simulink model "QPSK_short_4_tx_with_interference"  (R2023a)
settings: Solver=FixedStepAuto  StartTime=0.0  StopTime=inf  RelTol=1e-3
values from neighbouring files (symbols this model uses):
  fs_noise = 2*0.3e6    (= 600000)    [init_parameters_4_tx.m]
  Tx_Antennas = phased.ULA('NumElements',4,'ElementSpacing',0.05,'ArrayAxis','y')    [init_parameters_4_tx.m]
undefined symbols (not defined in the file or in its folder): physconst, qpsktxrx
libraries: dspmathops x4, dspsrcs4 x4, simulink x3, phasedtxrxlib x3, commdigbbndpm3 x3, dspsigops x3, commrflib2 x2, phasedbflib x2, commrfcorlib x2, dspstat3 x2, commsequence2 x2, commsync2 x2
settings Model: SimulationMode=accelerator  Creator=memre  LastModifiedBy=memre
settings DebuggingCC: ParameterOverflowMsg=none  ParameterUnderflowMsg=error

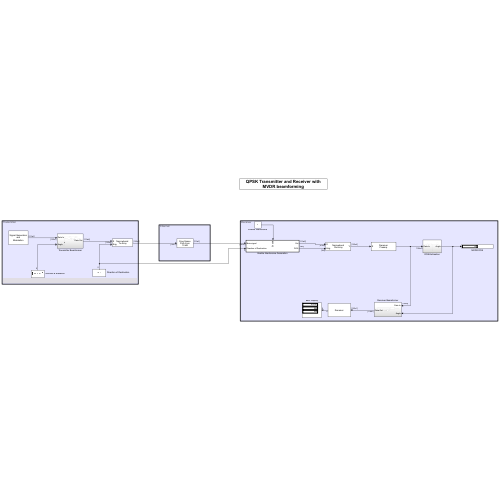
[thumbnail: Simulink's stored preview of the top-level diagram]
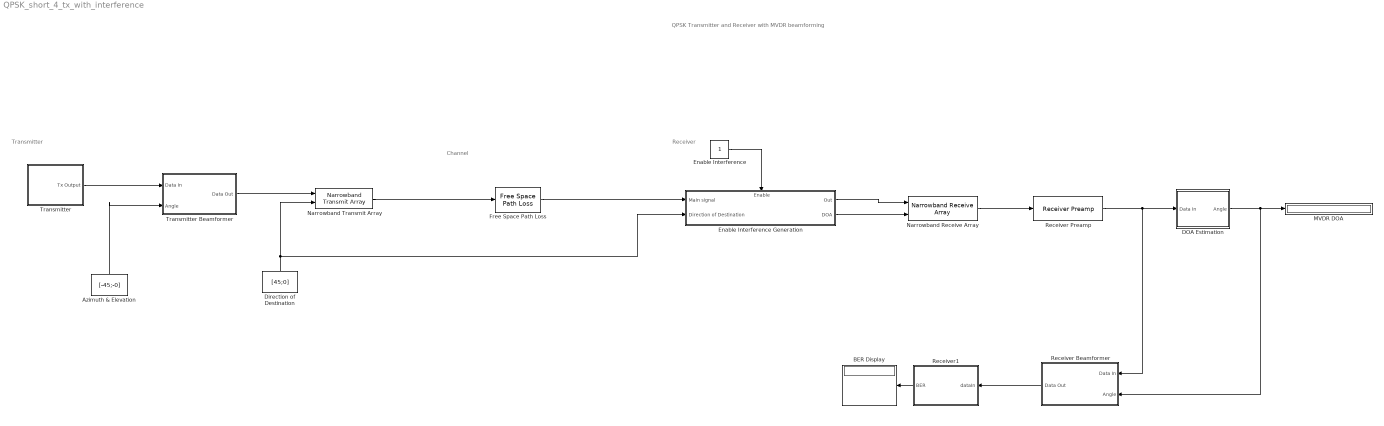
== system QPSK_short_4_tx_with_interference ==
  note: Receiver
  note: Transmitter
  note: Channel
  note: QPSK Transmitter and Receiver with MVDR beamforming
  Azimuth & Elevation : Constant  Value=[-45;-0]
  BER Display : Display
  DOA Estimation : Subsystem
  Direction of Destination : Constant  Value=[45;0]
  Enable Interference : Constant
  Enable Interference Generation : Subsystem  TreatAsAtomicUnit=on
      settings: PortSchema="{\"entries\":[{\"content\":{\"sides\":[{\"content\":{\"connectorIds\":[\"In1\",\"In2\"]},\"type\":\"ConnectorPlacement.EquallySpacedRectSide\",\"uuid\":\"34131771-bf07-4a9f-9b92-1cd845beac1b\"},{\"content\":{\"connectorIds\":[\"Out1\",\"Out2\"],\"side\":\"RIGHT\"},\"type\":\"ConnectorPlacement.EquallySpacedRectSide\",\"uuid\":\"139290bf-3e69-441d-8c76-d9406655bece\"},{\"content\":{\"connectorIds\":[\"In3\"],\"side\":\"TOP\"},\"type\":\"ConnectorPlacement.EquallySpacedRectSide\",\"uuid\":\"20149619-9d5d-4f55-89c0-ec473a07d659\"}]},\"type\":\"ConnectorPlacement.EquallySpacedConnector\",\"uuid\":\"f87a52e8-a08c-4e06-bc9a-bfdf8366a36e\"}],\"packageUris\":[\"http://schema.mathworks.com/mf0/Connector/R2020b\"],\"version\":\"1.0\"}"
  Free Space Path Loss : commrflib2/Free Space Path Loss  mode=Decibels  dB=10  d=0.100  fc=1920
  MVDR DOA : Display
  Narrowband Receive Array : phasedtxrxlib/Narrowband Receive Array  PropagationSpeed=prop_speed  OperatingFrequency=fc  Wavefront=Plane  SensorGainMeasure=dB  Polarization=None  WeightsInputPort=off  SimulateUsing=Interpreted execution  Sensor=Rx_Antennas
  Narrowband Transmit Array : phasedtxrxlib/Narrowband Transmit Array  PropagationSpeed=physconst( 'LightSpeed' )  OperatingFrequency=fc  CombineRadiatedSignals=on  SensorGainMeasure=dB  Polarization=None  WeightsInputPort=off  SimulateUsing=Code generation  Sensor=Tx_Antennas
  Receiver Beamformer : Subsystem
  Receiver Preamp : phasedtxrxlib/Receiver Preamp  Gain=0  LossFactor=0  NoiseMethod=Noise power  NoiseFigure=0  ReferenceTemperature=290  SampleRateFromInputCheckbox=on  SampleRate=1e6  NoisePower=.01  EnableInputPort=off  PhaseNoiseInputPort=off  SeedSource=Auto  Seed=0  SimulateUsing=Interpreted execution
  Receiver1 : Subsystem
      mask Display: disp('Receiver')
  Transmitter : Subsystem
      mask Display: disp('Signal Generation\nand\nModulation')
  Transmitter Beamformer : Subsystem
  wires:
  Receiver1/1(BER) -> BER Display/1
  Direction of Destination/1 -> Enable Interference Generation/2(Direction of Destination), Narrowband Transmit Array/2
  Narrowband Transmit Array/1 -> Free Space Path Loss/1
  Narrowband Receive Array/1 -> Receiver Preamp/1
  Receiver Preamp/1 -> Receiver Beamformer/1(Data In), DOA Estimation/1(Data In)
  Free Space Path Loss/1 -> Enable Interference Generation/1(Main signal)
  Enable Interference/1 -> Enable Interference Generation/3(Enable)
  Enable Interference Generation/1(Out) -> Narrowband Receive Array/1
  Enable Interference Generation/2(DOA) -> Narrowband Receive Array/2
  Transmitter/1(Tx Output) -> Transmitter Beamformer/1(Data In)
  Azimuth & Elevation/1 -> Transmitter Beamformer/2(Angle)
  Transmitter Beamformer/1(Data Out) -> Narrowband Transmit Array/1
  DOA Estimation/1(Angle) -> Receiver Beamformer/2(Angle), MVDR DOA/1
  Receiver Beamformer/1(Data Out) -> Receiver1/1(dataIn)

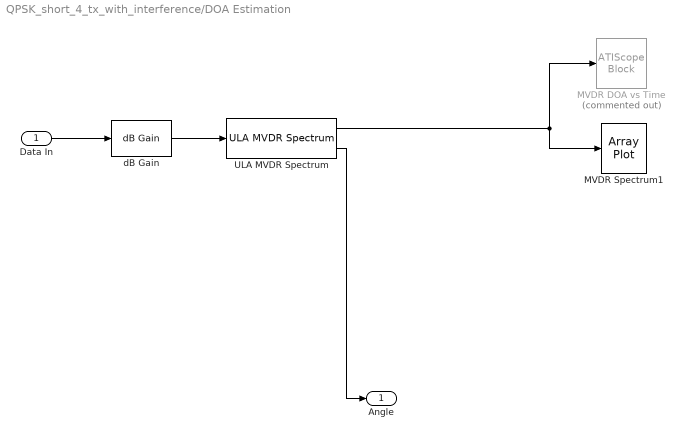
== system QPSK_short_4_tx_with_interference/DOA Estimation ==
  Data In : Inport
  MVDR DOA vs Time : ATIScopeBlock  Commented=on  WindowPosition=[64.000000,127.000000,669.000000,551.000000,]  ScopeFrameLocation=window  AngleLabel=Azimuth Angles (degree)  Title=Angle of Arrival vs. Time  TimeSpan=600  TimeResolution=0.3  ColorbarLabel=magnitude (V)  TimeResolutionSource=Property  TimeSpanSource=Property
  MVDR Spectrum1 : ArrayPlot  WindowPosition=[121.000000,272.000000,887.000000,614.000000,]  ScopeFrameLocation=window  XOffset=10  PlotType=Line  AxesScaling=Manual  Title=MVDR Spectrum  XLabel=Angle (degrees)  YLabel=Magnitude  YLimits=[-1,10]  ShowLegend=on  DefaultConfigurationName=dsp.scopes.ArrayPlotBlockSpecification
  ULA MVDR Spectrum : phaseddoalib/ULA MVDR Spectrum  PropagationSpeed=prop_speed  OperatingFrequency=fc  NumPhaseShifterBits=0  ForwardBackwardAveraging=off  SpatialSmoothing=0  ScanAngles=-90:90  DOAOutputPort=on  NumSignals=1  SimulateUsing=Interpreted execution  SensorArray=Rx_Antennas
  dB Gain : dspmathops/dB Gain  dB=20  intype=Amplitude
  Angle : Outport
  wires:
  ULA MVDR Spectrum/2 -> Angle/1
  ULA MVDR Spectrum/1 -> MVDR Spectrum1/1, MVDR DOA vs Time/1
  Data In/1 -> dB Gain/1
  dB Gain/1 -> ULA MVDR Spectrum/1

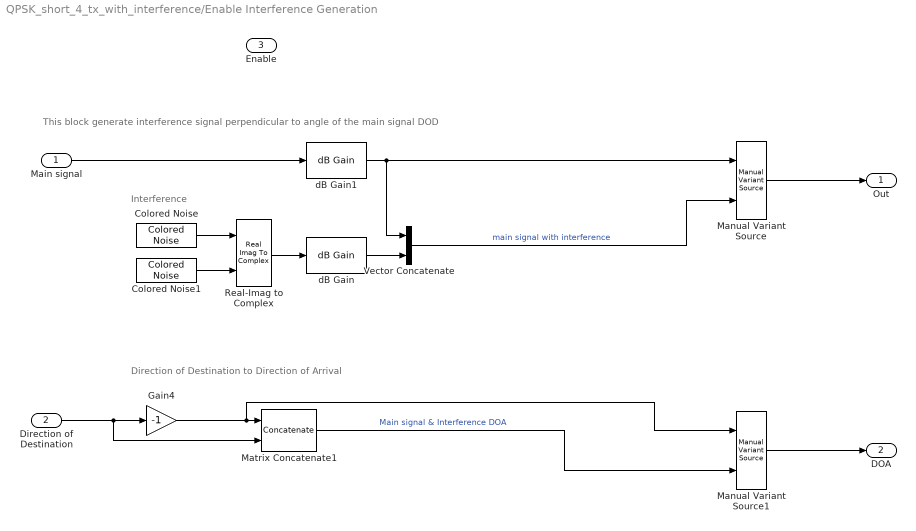
== system QPSK_short_4_tx_with_interference/Enable Interference Generation ==
  note: This block generate interference signal perpendicular to angle of the main signal DOD
  note: Interference
  note: Direction of Destination to Direction of Arrival
  Main signal : Inport
  Direction of Destination : Inport  Port=2
  Enable : Inport  Port=3
  Colored Noise : dspsrcs4/Colored Noise  Color=white  InverseFrequencyPower=1  BoundedOutput=on  NumChannels=1  OutputDataType=double  SamplesPerFrame=qpsktxrx.MessageLength * 7 * qpsktxrx.NumberOfMessage + qpsktxrx.HeaderLength  SampleTime=1/fs_noise  RandomStream=mt19937ar with seed  Seed=67  SimulateUsing=Code generation
  Colored Noise1 : dspsrcs4/Colored Noise  Color=white  InverseFrequencyPower=1  BoundedOutput=on  NumChannels=1  OutputDataType=double  SamplesPerFrame=qpsktxrx.MessageLength * 7 * qpsktxrx.NumberOfMessage + qpsktxrx.HeaderLength  SampleTime=1/fs_noise  RandomStream=mt19937ar with seed  Seed=32  SimulateUsing=Code generation
  Gain4 : Gain  Gain=-1
  Manual Variant Source : simulink/Signal Routing/Manual Variant Source  NumChoices=2  LabelModeActiveChoice=V_2
  Manual Variant Source1 : simulink/Signal Routing/Manual Variant Source  NumChoices=2  LabelModeActiveChoice=V_2
  Matrix Concatenate1 : Concatenate  Mode=Multidimensional array  ConcatenateDimension=2
  Real-Imag to Complex : RealImagToComplex
  Vector Concatenate : Concatenate  Mode=Multidimensional array  ConcatenateDimension=2
  dB Gain : dspmathops/dB Gain  dB=-10  intype=Amplitude
  dB Gain1 : dspmathops/dB Gain  dB=35  intype=Amplitude
  Out : Outport
  DOA : Outport  Port=2
  wires:
  Direction of Destination/1 -> Matrix Concatenate1/2, Gain4/1
  Colored Noise1/1 -> Real-Imag to Complex/2
  Colored Noise/1 -> Real-Imag to Complex/1
  Manual Variant Source/1 -> Out/1
  Manual Variant Source1/1 -> DOA/1
  Gain4/1 -> Manual Variant Source1/1, Matrix Concatenate1/1
  Vector Concatenate/1 -> Manual Variant Source/2  "main signal with interference"
  Real-Imag to Complex/1 -> dB Gain/1
  dB Gain/1 -> Vector Concatenate/2
  dB Gain1/1 -> Manual Variant Source/1, Vector Concatenate/1
  Main signal/1 -> dB Gain1/1
  Matrix Concatenate1/1 -> Manual Variant Source1/2  "Main signal & Interference DOA"

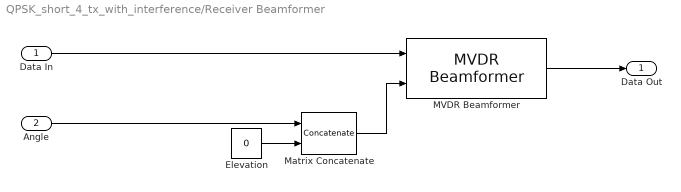
== system QPSK_short_4_tx_with_interference/Receiver Beamformer ==
  Data In : Inport
  Angle : Inport  Port=2
  Elevation : Constant  Value=0
  MVDR Beamformer : phasedbflib/MVDR Beamformer  PropagationSpeed=prop_speed  OperatingFrequency=fc  DiagonalLoadingFactor=0  TrainingInputPort=off  DirectionSource=Input port  Direction=DOA  NumPhaseShifterBits=0  WeightsOutputPort=off  SimulateUsing=Interpreted execution  SensorArray=Rx_Antennas
  Matrix Concatenate : Concatenate  ConcatenateDimension=2
  Data Out : Outport
  wires:
  Angle/1 -> Matrix Concatenate/1
  Matrix Concatenate/1 -> MVDR Beamformer/2
  Elevation/1 -> Matrix Concatenate/2
  MVDR Beamformer/1 -> Data Out/1
  Data In/1 -> MVDR Beamformer/1

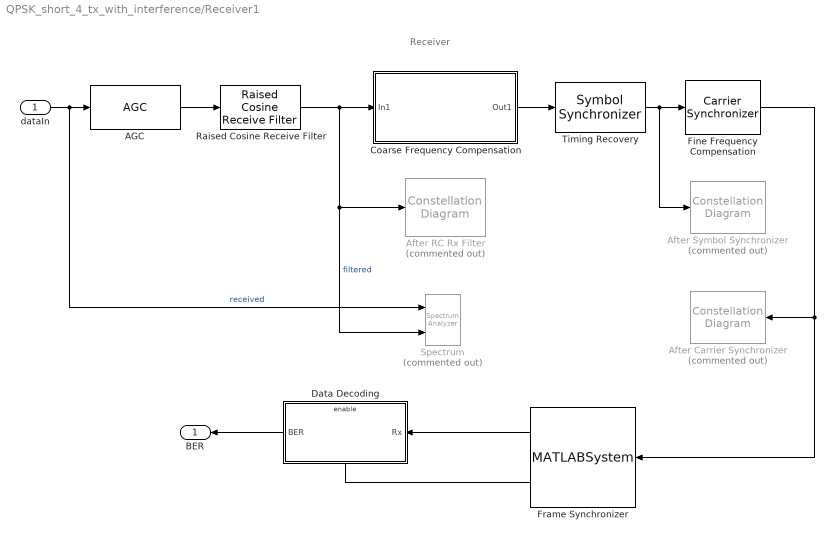
== system QPSK_short_4_tx_with_interference/Receiver1 ==
  note: Receiver
  dataIn : Inport
  AGC : commrfcorlib/AGC  LegacyMode=off  DetectorMethod=Rectifier  LoopMethod=Linear  UpdatePeriod=100  StepSize=0.1  AdaptationStepSize=0.01  DesiredOutputPower=qpsktxrx.DesiredPower  AveragingLength=qpsktxrx.AveragingLength  MaximumGain=30  MaxPowerGain=qpsktxrx.MaxPowerGain  GainOutputPort=off  InputPowerOutputPort=off  SimulateUsing=Code generation
  After Carrier Synchronizer : ConstellationDiagram  Tag=ScatterPlot  Commented=on  WindowPosition=[668.000000,189.000000,534.000000,257.000000,]  ScopeFrameLocation=window  SamplesPerSymbol=qpsktxrx.Interpolation  SymbolsToDisplaySource=Property  SymbolsToDisplay=qpsktxrx.FrameSize  ReferenceConstellation=QPSK  Title=After Carrier Synchronizer  XLimits=[-3 3]  YLimits=[-3 3]  EnableMeasurements=on  DefaultConfigurationName=comm.scopes.ConstellationDiagramBlockCfg
  After RC Rx Filter : ConstellationDiagram  Tag=ScatterPlot  Commented=on  WindowPosition=[66.000000,211.000000,260.000000,258.000000,]  ScopeFrameLocation=window  SamplesPerSymbol=qpsktxrx.Interpolation  SymbolsToDisplaySource=Property  SymbolsToDisplay=qpsktxrx.FrameSize  ReferenceConstellation=QPSK  Title=After Raised Cosine Rx Filter  XLimits=[-3.1734 3.2134]  YLimits=[-3.1734 3.2134]  DefaultConfigurationName=comm.scopes.ConstellationDiagramBlockCfg
  After Symbol Synchronizer : ConstellationDiagram  Tag=ScatterPlot  Commented=on  WindowPosition=[351.000000,211.000000,284.000000,258.000000,]  ScopeFrameLocation=window  SamplesPerSymbol=2  SymbolsToDisplaySource=Property  SymbolsToDisplay=qpsktxrx.FrameSize  ReferenceConstellation=QPSK  Title=After Symbol Synchronizer  XLimits=[-3.0085 2.9872]  YLimits=[-3.0085 2.9872]  DefaultConfigurationName=comm.scopes.ConstellationDiagramBlockCfg
  Coarse Frequency Compensation : Subsystem
      mask Display: fprintf('Coarse Frequency\nCompensation')
  Data Decoding : Subsystem
      mask Display: disp('Data Decoding');
  Fine Frequency Compensation : commsync2/Carrier Synchronizer  Modulation=QPSK  ModulationPhaseOffset=Auto  CustomPhaseOffset=0  SamplesPerSymbol=qpsktxrx.Interpolation/qpsktxrx.Decimation  DampingFactor=1  NormalizedLoopBandwidth=0.01  EstimatedPhaseErrorOutputPort=off  SimulateUsing=Code generation
  Frame Synchronizer : MATLABSystem  System=FrameSynchronizer  Preamble=sqrt(2)/2 * (-1-1i) * (qpsktxrx.BarkerCode)'  Threshold=qpsktxrx.PreambleDetectionThreshold  OutputLength=qpsktxrx.FrameSize  SimulateUsing=Code generation
      mask Type: FrameSynchronizer
      mask Display:
      | disp(['Frame' char(10) 'Synchronizer']);
      | port_label('input',1,'x');
      | port_label('output',1,'Frame');
      | port_label('output',2,'Valid');
  Raised Cosine Receive Filter : commfilt2/Raised Cosine Receive Filter  filtType=Square root  R=qpsktxrx.RolloffFactor  filtSpan=qpsktxrx.RaisedCosineFilterSpan  N=qpsktxrx.Interpolation  downFactor=qpsktxrx.Decimation  downOffset=0  filterGain=1  InputProcessing=Columns as channels (frame based)  RateOptions=Enforce single-rate processing  framing=Mute  checkCoeff=off  variableName=rcRxFilt  currentFiltSpan=10  D=5  inputOffset=0  sampMode=Mute  saveAsFlag=0  rateMode=Downsampling  checkGain=Normalized  launchFVT=on  roundingMode=Floor  overflowMode=off  coeffDataTypeStr=Inherit: Same word length as input  coeffMin=[]  coeffMax=[]  coeffLastDataTypeStr=Inherit: Same word length as input  accumDataTypeStr=Inherit: Same as product output  accumLastDataTypeStr=Inherit: Same as product output  outputDataTypeStr=Inherit: Same as accumulator  outputMin=[]  outputMax=[]  outputLastDataTypeStr=Inherit: Same as accumulator
  Spectrum : SpectrumAnalyzer  Commented=on  NumInputPorts=2  WindowPosition=[1155.000000,275.000000,800.000000,500.000000,]  ScopeFrameLocation=window  Method=Welch  SampleRate=100000  AxesScaling=Manual  Span=100000  StartFrequency=-50000  StopFrequency=50000  RBWSource=Property  RBW=75  FFTLength=128  AveragingMethod=Running  SpectralAverages=2  SpectrumUnits=dBW  Title=After Raised Cosine Rx Filter  YLabel=Power Spectrum  YLimits=[-137.6344738236879266 40]  ShowLegend=on
  Timing Recovery : commsync2/Symbol Synchronizer  Modulation=PAM/PSK/QAM  TimingErrorDetector=Gardner (non-data-aided)  SamplesPerSymbol=qpsktxrx.Interpolation/qpsktxrx.Decimation  DampingFactor=1  NormalizedLoopBandwidth=0.01  DetectorGain=qpsktxrx.TimingErrorDetectorGain  TimingErrorOutputPort=off  SimulateUsing=Code generation
  BER : Outport  VectorParamsAs1DForOutWhenUnconnected=off
  wires:
  Raised Cosine Receive Filter/1 -> Coarse Frequency Compensation/1(In1), Spectrum/2, After RC Rx Filter/1  "filtered"
  dataIn/1 -> Spectrum/1, AGC/1  "received"
  AGC/1 -> Raised Cosine Receive Filter/1
  Fine Frequency Compensation/1 -> Frame Synchronizer/1, After Carrier Synchronizer/1
  Frame Synchronizer/1 -> Data Decoding/1(Rx)
  Data Decoding/1(BER) -> BER/1
  Frame Synchronizer/2 -> Data Decoding/Enable
  Coarse Frequency Compensation/1(Out1) -> Timing Recovery/1
  Timing Recovery/1 -> After Symbol Synchronizer/1, Fine Frequency Compensation/1

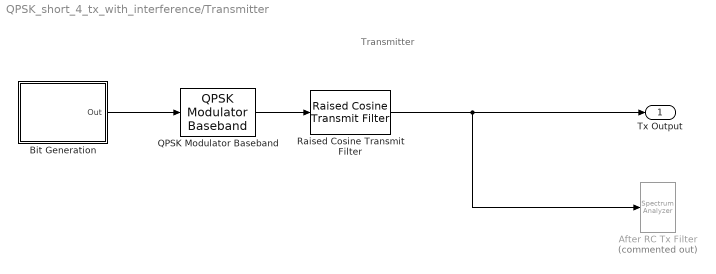
== system QPSK_short_4_tx_with_interference/Transmitter ==
  note: Transmitter
  After RC Tx Filter : SpectrumAnalyzer  Commented=on  Method=Welch  SampleRate=200000  Span=200000  StartFrequency=-100000  StopFrequency=100000  RBWSource=Property  RBW=750  FFTLength=128  AveragingMethod=Running  SpectralAverages=2  SpectrumUnits=dBW  YLabel=Spectrum after Raised-Cosine Tx Filter  YLimits=[-114.15736879359562 -6.4493918406395565]
      settings: OpenAtSimulationStart=off
  Bit Generation : Subsystem
      mask Display: disp('Bits Generation')
  QPSK Modulator Baseband : commdigbbndpm3/QPSK Modulator Baseband  InType=Bit  Enc=Gray  Ph=pi/4  outDtype=double  outWordLen=16  outUDDataType=sfix(16)  outFracLenMode=Best precision  outFracLen=15  outDataTypeStr=double  outLastDataTypeStr=double
  Raised Cosine Transmit Filter : commfilt2/Raised Cosine Transmit Filter  filtType=Square root  R=qpsktxrx.RolloffFactor  filtSpan=qpsktxrx.RaisedCosineFilterSpan  N=qpsktxrx.Interpolation  filterGain=1  InputProcessing=Columns as channels (frame based)  RateOptions=Enforce single-rate processing  framing=Mute  checkCoeff=off  variableName=rcTxFilt1  checkGain=Normalized  sampMode=Mute  saveAsFlag=0  currentFiltSpan=10  D=5  launchFVT=on  roundingMode=Floor  overflowMode=off  coeffDataTypeStr=Inherit: Same word length as input  coeffMin=[]  coeffMax=[]  coeffLastDataTypeStr=Inherit: Same word length as input  outputDataTypeStr=Inherit: Same as accumulator  outputMin=[]  outputMax=[]  outputLastDataTypeStr=Inherit: Same as accumulator
  Tx Output : Outport  VectorParamsAs1DForOutWhenUnconnected=off
  wires:
  QPSK Modulator Baseband/1 -> Raised Cosine Transmit Filter/1
  Bit Generation/1(Out) -> QPSK Modulator Baseband/1
  Raised Cosine Transmit Filter/1 -> Tx Output/1, After RC Tx Filter/1

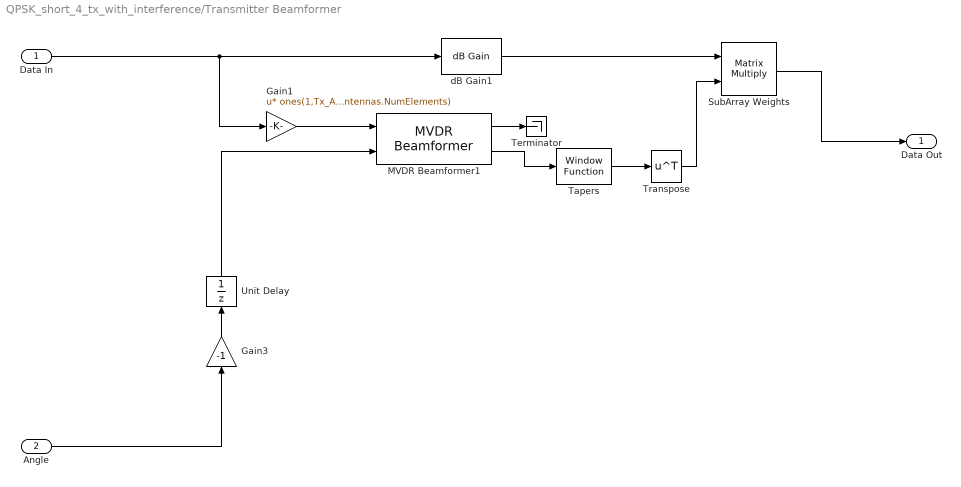
== system QPSK_short_4_tx_with_interference/Transmitter Beamformer ==
  Data In : Inport
  Angle : Inport  Port=2
  Gain1 : Gain  Gain=ones(1,Tx_Antennas.NumElements)  Multiplication=Matrix(u*K)
  Gain3 : Gain  Gain=-1
  MVDR Beamformer1 : phasedbflib/MVDR Beamformer  PropagationSpeed=prop_speed  OperatingFrequency=fc  DiagonalLoadingFactor=0.1  TrainingInputPort=off  DirectionSource=Input port  Direction=DOA  NumPhaseShifterBits=0  WeightsOutputPort=on  SimulateUsing=Code generation  SensorArray=Tx_Antennas
  SubArray Weights : Product  Multiplication=Matrix(*)
  Tapers : dspsigops/Window Function  winmode=Apply window to input  wintype=Hamming  sampmode=Continuous  samptime=1  N=64  Rs=50  beta=10  winsamp=Symmetric  UserWindow=hamming  OptParams=off  UserParams={'symmetric'}  dataType=double  isSigned=on  wordLen=16  udDataType=sfix(16)  fracBitsMode=Best precision  numFracBits=15  roundingMode=Floor  overflowMode=off  numSidelobes=4  sidelobeLevel=-30
  Terminator : Terminator
  Transpose : Math  Operator=transpose
  Unit Delay : UnitDelay  SampleTime=-1  HasFrameUpgradeWarning=on
  dB Gain1 : dspmathops/dB Gain  dB=0  intype=Amplitude
  Data Out : Outport
  wires:
  Transpose/1 -> SubArray Weights/2
  dB Gain1/1 -> SubArray Weights/1
  MVDR Beamformer1/1 -> Terminator/1
  MVDR Beamformer1/2 -> Tapers/1
  SubArray Weights/1 -> Data Out/1
  Tapers/1 -> Transpose/1
  Data In/1 -> dB Gain1/1, Gain1/1
  Gain3/1 -> Unit Delay/1
  Unit Delay/1 -> MVDR Beamformer1/2
  Gain1/1 -> MVDR Beamformer1/1
  Angle/1 -> Gain3/1

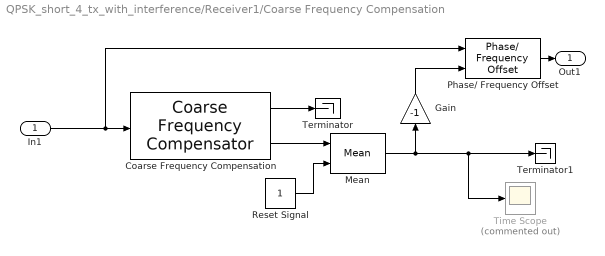
== system QPSK_short_4_tx_with_interference/Receiver1/Coarse Frequency Compensation ==
  In1 : Inport
  Coarse Frequency Compensation : commrfcorlib/Coarse Frequency Compensator  Modulation=QPSK  Algorithm=Correlation-based  FrequencyResolution=25  MaximumFrequencyOffset=12.5e3  SamplesPerSymbol=4  EstimatedFreqOffsetPort=on  SimulateUsing=Code generation
  Gain : Gain  Gain=-1
  Mean : dspstat3/Mean  run=on  InputProcessing=Columns as channels (frame based)  reset_popup=Either edge  directionMode=Each column  dimension=1  roiEnable=off  roiType=Rectangles  roiPortion=Entire ROI  roiOutput=Individual statistics for each ROI  roiFlag=off  roundingMode=Floor  overflowMode=off  outputDataTypeStr=Inherit: Same as accumulator  outputMin=[]  outputMax=[]  outputLastDataTypeStr=Inherit: Same as accumulator
  Phase/ Frequency Offset : commrflib2/Phase// Frequency Offset  phaseOffset=0  freqPort=on  freqOffset=0
  Reset Signal : Constant
  Terminator : Terminator
  Terminator1 : Terminator
  Time Scope : Scope  Commented=on
  Out1 : Outport  VectorParamsAs1DForOutWhenUnconnected=off
  wires:
  In1/1 -> Phase/ Frequency Offset/1, Coarse Frequency Compensation/1
  Phase/ Frequency Offset/1 -> Out1/1
  Mean/1 -> Time Scope/1, Terminator1/1, Gain/1
  Coarse Frequency Compensation/2 -> Mean/1
  Coarse Frequency Compensation/1 -> Terminator/1
  Gain/1 -> Phase/ Frequency Offset/2
  Reset Signal/1 -> Mean/2

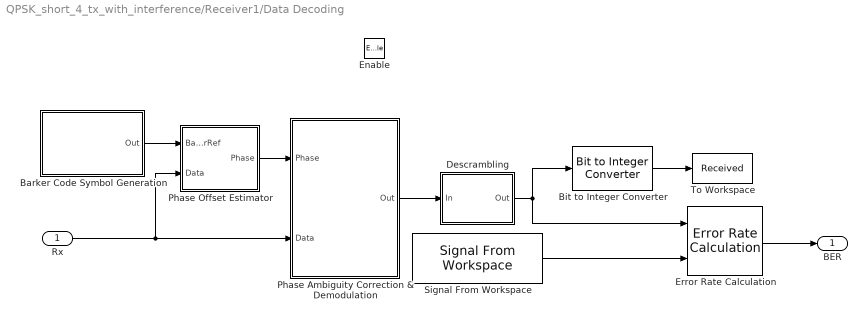
== system QPSK_short_4_tx_with_interference/Receiver1/Data Decoding ==
  Rx : Inport
  Enable : EnablePort
  "Barker Code Symbol Generation " : Subsystem
      mask Display: disp('Barker Code\nSymbol Generation')
  Bit to Integer Converter : simulink/Logic and Bit Operations/Bit to Integer Converter  nbits=7  bitOrder=MSB first  signedOutputValues=Unsigned  outDtype=Inherit via internal rule  outDtypeSigned=Inherit via internal rule
  Descrambling : Subsystem
      mask Display: disp('Descrambling');
  Error Rate Calculation : commsink2/Error Rate Calculation  N=0  st_delay=0  cp_mode=Select samples from mask  subframe=qpsktxrx.BerMask  PMode=Port  WsName=ErrorVec  RsMode2=off  stop=off  numErr=100  maxBits=1e6
  Phase Ambiguity Correction & Demodulation : Subsystem
      mask Display: disp('Phase Ambiguity\nCorrection\n& Demodulation');
  Phase Offset Estimator : Subsystem
  Signal From Workspace : dspsrcs4/Signal From Workspace  X=qpsktxrx.MessageBits  Ts=1/qpsktxrx.PayloadLength*qpsktxrx.FrameTime  nsamps=qpsktxrx.MessageLength * 7 * qpsktxrx.NumberOfMessage  OutputAfterFinalValue=Cyclic repetition  ignoreOrWarnInputAndFrameLengths=off  OutputFrames=off
  To Workspace : ToWorkspace  VariableName=Received  SaveFormat=Structure  SampleTime=-1
      settings: Save2DSignal=2-D array (concatenate along first dimension)
  BER : Outport  VectorParamsAs1DForOutWhenUnconnected=off
  wires:
  "Barker Code Symbol Generation "/1(Out) -> Phase Offset Estimator/1(BarkerRef)
  Phase Offset Estimator/1(Phase) -> Phase Ambiguity Correction & Demodulation/1(Phase)
  Rx/1 -> Phase Offset Estimator/2(Data), Phase Ambiguity Correction & Demodulation/2(Data)
  Descrambling/1(Out) -> Error Rate Calculation/1, Bit to Integer Converter/1
  Error Rate Calculation/1 -> BER/1
  Phase Ambiguity Correction & Demodulation/1(Out) -> Descrambling/1(In)
  Signal From Workspace/1 -> Error Rate Calculation/2
  Bit to Integer Converter/1 -> To Workspace/1

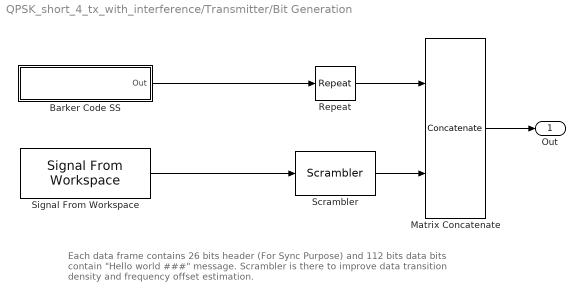
== system QPSK_short_4_tx_with_interference/Transmitter/Bit Generation ==
  note: Each data frame contains 26 bits header (For Sync Purpose) and 112 bits data bits
      | contain "Hello world ###" message. Scrambler is there to improve data
      | transition density and frequency offset estimation.
  Barker Code SS : Subsystem
      mask Display: disp('Unipolar\nBarker Code')
  Matrix Concatenate : Concatenate  Mode=Multidimensional array
  Repeat : dspsigops/Repeat  FactorSource=Dialog parameter  N=2  Nmax=16  InputProcessing=Columns as channels (frame based)  RateOptions=Enforce single-rate processing  ic=0  mode=Unused parameter value
  Scrambler : commsequence2/Scrambler  M=2  poly=[1 1 1 0 1]  iniStaSource=Dialog Parameter  ini_sta=[0 0 0 0]  resetViaPort=off
  Signal From Workspace : dspsrcs4/Signal From Workspace  X=qpsktxrx.MessageBits  Ts=1/qpsktxrx.PayloadLength*qpsktxrx.FrameTime  nsamps=qpsktxrx.MessageLength * 7 * qpsktxrx.NumberOfMessage  OutputAfterFinalValue=Cyclic repetition  ignoreOrWarnInputAndFrameLengths=off  OutputFrames=off
  Out : Outport  VectorParamsAs1DForOutWhenUnconnected=off
  wires:
  Barker Code SS/1(Out) -> Repeat/1
  Matrix Concatenate/1 -> Out/1
  Repeat/1 -> Matrix Concatenate/1
  Scrambler/1 -> Matrix Concatenate/2
  Signal From Workspace/1 -> Scrambler/1

== system QPSK_short_4_tx_with_interference/Receiver1/Data Decoding/Barker Code Symbol Generation  ==
  note: Regenerate a QPSK-modulated unipolar Barker code sequence
      | to be compared with the received data
  Constant Barker Code : Constant  Value=(qpsktxrx.BarkerCode)' > 0  VectorParams1D=off  OutDataTypeStr=double
  QPSK Modulator Baseband : commdigbbndpm3/QPSK Modulator Baseband  InType=Bit  Enc=Gray  Ph=pi/4  outDtype=double  outWordLen=16  outUDDataType=sfix(16)  outFracLenMode=Best precision  outFracLen=15  outDataTypeStr=double  outLastDataTypeStr=double
  Repeat : dspsigops/Repeat  FactorSource=Dialog parameter  N=2  Nmax=16  InputProcessing=Columns as channels (frame based)  RateOptions=Enforce single-rate processing  ic=0  mode=Unused parameter value
  Out : Outport  VectorParamsAs1DForOutWhenUnconnected=off
  wires:
  Constant Barker Code/1 -> Repeat/1
  Repeat/1 -> QPSK Modulator Baseband/1
  QPSK Modulator Baseband/1 -> Out/1

== system QPSK_short_4_tx_with_interference/Receiver1/Data Decoding/Descrambling ==
  In : Inport
  Descrambler : commsequence2/Descrambler  M=2  poly=[1 1 1 0 1]  iniStaSource=Dialog Parameter  ini_sta=[0 0 0 0]  resetViaPort=off
  Selector : Selector  IndexOptions=Index vector (dialog)  Indices=[qpsktxrx.HeaderLength+(1 : qpsktxrx.PayloadLength)]  OutputSizes=1
  Out : Outport  VectorParamsAs1DForOutWhenUnconnected=off
  wires:
  In/1 -> Selector/1
  Selector/1 -> Descrambler/1
  Descrambler/1 -> Out/1

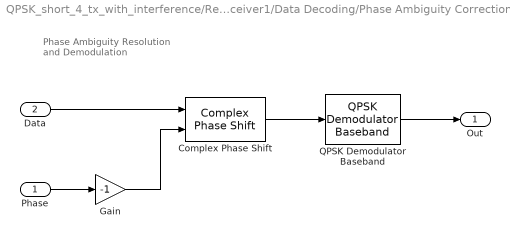
== system QPSK_short_4_tx_with_interference/Receiver1/Data Decoding/Phase Ambiguity Correction & Demodulation ==
  note: Phase Ambiguity Resolution
      | and Demodulation
  Phase : Inport
  Data : Inport  Port=2
  Complex Phase Shift : commutil2/Complex Phase Shift
  Gain : Gain  Gain=-1  OutDataTypeStr=Inherit: Same as input
  QPSK Demodulator Baseband : commdigbbndpm3/QPSK Demodulator Baseband  OutType=Bit  DecType=Hard decision  VarSource=Dialog  Variance=1  Dec=Gray  Ph=pi/4  outDtype1=Inherit via internal rule  outDtype2=Inherit via internal rule  derotateFactorWordLen=16  derotateFactorDataTypeStr=Inherit: Same word length as input  derotateFactorLastDataTypeStr=Inherit: Same word length as input
  Out : Outport  VectorParamsAs1DForOutWhenUnconnected=off
  wires:
  Phase/1 -> Gain/1
  Data/1 -> Complex Phase Shift/1
  Complex Phase Shift/1 -> QPSK Demodulator Baseband/1
  QPSK Demodulator Baseband/1 -> Out/1
  Gain/1 -> Complex Phase Shift/2

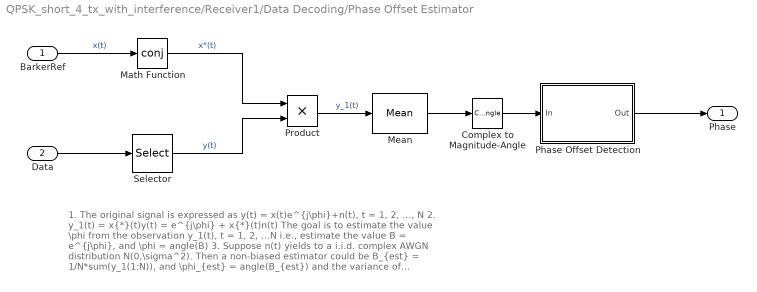
== system QPSK_short_4_tx_with_interference/Receiver1/Data Decoding/Phase Offset Estimator ==
  note: 1. The original signal is expressed as y(t) = x(t)e^{j\phi}+n(t), t = 1, 2, ..., N
      | 2. y_1(t) = x{*}(t)y(t) = e^{j\phi} + x{*}(t)n(t)
      | The goal is to estimate the value \phi from the observation y_1(t), t = 1, 2, ...N
      | i.e., estimate the value B = e^{j\phi}, and \phi = angle(B)
      | 3. Suppose n(t) yields to a i.i.d. complex AWGN distribution N(0,\sigma^2).
      | Then a non-biased estimator could be
      | B_{est} = 1/N*sum(y_1(1:N)), and \phi_{est} = angle(B_{est})
      | and the variance of B_{est} is \sigma^2/N
  BarkerRef : Inport
  Data : Inport  Port=2
  Complex to Magnitude-Angle : ComplexToMagnitudeAngle  Output=Angle
  Math Function : Math  Operator=conj  SignedPower=on
  Mean : dspstat3/Mean  run=off  InputProcessing=Columns as channels (frame based)  reset_popup=None  directionMode=Each column  dimension=1  roiEnable=off  roiType=Rectangles  roiPortion=Entire ROI  roiOutput=Individual statistics for each ROI  roiFlag=off  roundingMode=Floor  overflowMode=off  outputDataTypeStr=Inherit: Same as accumulator  outputMin=[]  outputMax=[]  outputLastDataTypeStr=Inherit: Same as accumulator
  Phase Offset Detection : MATLAB Function  TreatAsAtomicUnit=on
  Product : Product  RndMeth=Zero
  Selector : Selector  IndexOptions=Index vector (dialog)  Indices=[1:qpsktxrx.BarkerLength]  OutputSizes=1
  Phase : Outport  VectorParamsAs1DForOutWhenUnconnected=off
  wires:
  Data/1 -> Selector/1
  BarkerRef/1 -> Math Function/1  "x(t)"
  Selector/1 -> Product/2  "y(t)"
  Math Function/1 -> Product/1  "x*(t)"
  Product/1 -> Mean/1  "y_1(t)"
  Mean/1 -> Complex to Magnitude-Angle/1
  Complex to Magnitude-Angle/1 -> Phase Offset Detection/1(In)
  Phase Offset Detection/1(Out) -> Phase/1

== system QPSK_short_4_tx_with_interference/Transmitter/Bit Generation/Barker Code SS ==
  Constant Barker Code : Constant  Value=(qpsktxrx.BarkerCode)' > 0; % Bipolar to Unipolar  VectorParams1D=off  OutDataTypeStr=double
  Out : Outport  VectorParamsAs1DForOutWhenUnconnected=off
  wires:
  Constant Barker Code/1 -> Out/1

== matlab function QPSK_short_4_tx_with_interference/Receiver1/Data Decoding/Phase Offset Estimator/Phase Offset Detection ==
  data: In input; Out output
function Out = phasedecision(In)
% Map the estimated phase to one of -pi, -pi/2, 0, pi/2,  
%#codegen
Out = round(In.*2./pi)./2.*pi;
% The above processing is equivalent to the following processing using
% if/else statements
%
% if In<pi/4 && In>-pi/4
%     Out = 0;
% elseif In>=pi/4 && In<pi*3/4
%     Out = pi/2;
% elseif In>=pi*3/4 || In<=-pi*3/4
%     Out = -pi;
% else
%     Out = -pi/2;
% end
